simulink model "THRESHER_CONTROLLER_SIM"  (R2026a)
settings: Solver=FixedStepAuto  StopTime=500  FixedStep=0.05  EnableMultiTasking=on
undefined symbols (not defined in the file): A_ph, A_sy, Bsys_ph, Bsys_sy, C_ph, C_sy, DiscIntNeverNeededParam, GAMMA_ph, GAMMA_sy, K1_ph, K1_sy, K2_ph, K2_sy, L_ph, L_sy, PHI_ph, PHI_sy, T
settings Model: Creator=The MathWorks, Inc.  LastModifiedBy=env
settings OptimizationCC: PassReuseOutputArgsThreshold=0.0
settings HardwareCC: TargetHWDeviceType=Generic->Unspecified (assume 32-bit Generic)  UseEmbeddedCoderFeatures=off
settings SFSimCC: SimTargetLang=C++
settings RTWCC: SystemTargetFile=ert.tlc  HardwareBoard=Robot Operating System 2 (ROS 2)  TLCOptions="-aInlineSetEventsForThisBaseRateFcn=TLC_FALSE -aSuppressMultiTaskScheduler=TLC_FALSE  -aRateBasedStepFcn=0"  Toolchain=Colcon Tools  TargetLang=C++  Description=Embedded Coder
settings ERTTargetCC: ExtModeTransport=2.0  ExtModeAutomaticAllocSize=off  DynamicArrayContainerType=coder::array  ERTCustomFileBanners=off  CodeInterfacePackaging=C++ class  SupportContinuousTime=on  SupportNonInlinedSFcns=on  SupportVariableSizeSignals=on  ModelStepFunctionPrototypeControlCompliant=off

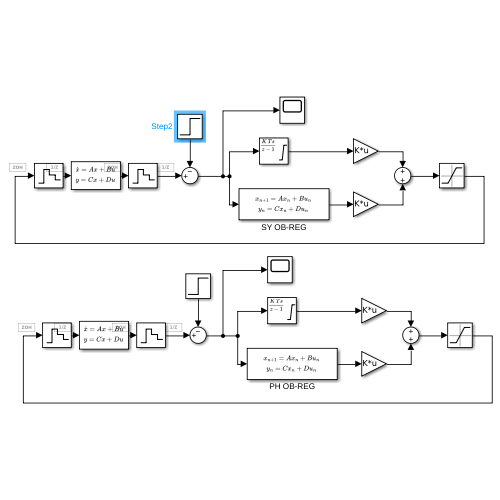
[thumbnail: Simulink's stored preview of the top-level diagram]
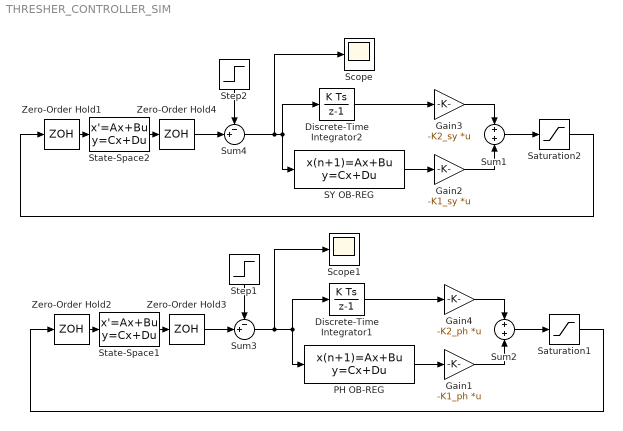
== system THRESHER_CONTROLLER_SIM ==
  Discrete-Time Integrator1 : DiscreteIntegrator  gainval=1  SampleTime=-1  LimitOutput=on  UpperSaturationLimit=(-pi/6)/K2_ph  LowerSaturationLimit=(pi/6)/K2_ph  ICPrevOutput=DiscIntNeverNeededParam  ICPrevScaledInput=DiscIntNeverNeededParam
  Discrete-Time Integrator2 : DiscreteIntegrator  gainval=1  SampleTime=-1  LimitOutput=on  UpperSaturationLimit=(pi/6)/K2_sy  LowerSaturationLimit=(-pi/6)/K2_sy  ICPrevOutput=DiscIntNeverNeededParam  ICPrevScaledInput=DiscIntNeverNeededParam
  Gain1 : Gain  Gain=-K1_ph  Multiplication=Matrix(K*u)
  Gain2 : Gain  Gain=-K1_sy  Multiplication=Matrix(K*u)
  Gain3 : Gain  Gain=-K2_sy  Multiplication=Matrix(K*u)
  Gain4 : Gain  Gain=-K2_ph  Multiplication=Matrix(K*u)
  PH OB-REG : DiscreteStateSpace  A=(PHI_ph-L_ph*C_ph-GAMMA_ph*K1_ph)  B=L_ph  C=eye(4)  D=zeros(4,1)  InitialCondition=[0;0;0;0]  SampleTime=-1
  SY OB-REG : DiscreteStateSpace  A=(PHI_sy-L_sy*C_sy-GAMMA_sy*K1_sy)  B=L_sy  C=eye(3)  D=zeros(3,1)  InitialCondition=[0;0;0]  SampleTime=-1
  Saturation1 : Saturate  UpperLimit=pi/6  LowerLimit=-pi/6
  Saturation2 : Saturate  UpperLimit=pi/6  LowerLimit=-pi/6
  Scope : Scope
      settings: ActiveDisplayYMinimum=-1  ActiveDisplayYMaximum=1
  Scope1 : Scope
      settings: ActiveDisplayYMinimum=-1  ActiveDisplayYMaximum=1
  State-Space1 : StateSpace  A=A_ph  B=Bsys_ph  C=C_ph  D=0  InitialCondition=0
  State-Space2 : StateSpace  A=A_sy  B=Bsys_sy  C=C_sy  D=0  InitialCondition=0
  Step1 : Step  Time=0  FinalValue=25  SampleTime=0
  Step2 : Step  Time=0  FinalValue=pi  SampleTime=0
  Sum1 : Sum  Inputs=+|+
  Sum2 : Sum  Inputs=+|+
  Sum3 : Sum  Inputs=-+|
  Sum4 : Sum  Inputs=-+|
  Zero-Order Hold{1..4} (4 alike) : ZeroOrderHold  SampleTime=T
  wires:
  PH OB-REG/1 -> Gain1/1
  Discrete-Time Integrator1/1 -> Gain4/1
  Gain1/1 -> Sum2/2
  Sum2/1 -> Saturation1/1
  State-Space1/1 -> Zero-Order Hold3/1
  Zero-Order Hold2/1 -> State-Space1/1
  Step1/1 -> Sum3/1
  Zero-Order Hold3/1 -> Sum3/2
  Sum3/1 -> Scope1/1, PH OB-REG/1, Discrete-Time Integrator1/1
  Saturation1/1 -> Zero-Order Hold2/1
  Zero-Order Hold1/1 -> State-Space2/1
  State-Space2/1 -> Zero-Order Hold4/1
  Saturation2/1 -> Zero-Order Hold1/1
  SY OB-REG/1 -> Gain2/1
  Sum4/1 -> Scope/1, SY OB-REG/1, Discrete-Time Integrator2/1
  Sum1/1 -> Saturation2/1
  Discrete-Time Integrator2/1 -> Gain3/1
  Gain2/1 -> Sum1/2
  Zero-Order Hold4/1 -> Sum4/2
  Step2/1 -> Sum4/1
  Gain3/1 -> Sum1/1
  Gain4/1 -> Sum2/1
